simulink model "SiMoDronesBebopRos_student"  (R2021a)
settings: Solver=FixedStepAuto  StartTime=0  StopTime=35  FixedStep=0.005  MaxStep=1e-3  MinStep=5e-5  RelTol=1e-5  AbsTol=1e-5
StopFcn:
  | %data_bebop;
  | save_and_plot_data
values from neighbouring files (symbols this model uses):
  aero =     [test1_p1.mat]    (also in test2_P2.mat; test3_pd.mat; test4_lat.mat; xtest4_lat.mat)
  controlGains =     [test1_p1.mat]    (also in test2_P2.mat; test3_pd.mat; test4_lat.mat; xtest4_lat.mat)
  drone =     [test1_p1.mat]    (also in test2_P2.mat; test3_pd.mat; test4_lat.mat; xtest4_lat.mat)
  init_state =     [test1_p1.mat]    (also in test2_P2.mat; test3_pd.mat; test4_lat.mat; xtest4_lat.mat)
  K = place(A,B,P0)    [Control.m]    (also in test1_p1.mat = [0.637104994903 0.356778797146]; test2_P2.mat = [0.637104994903 0.356778797146]; test3_pd.mat = [0.637104994903 0.356778797146]; test4_lat.mat = [0.637104994903 0.356778797146])
  Kd = 3.806    [Control.m]    (also in test1_p1.mat = 5.726; test2_P2.mat = 5.726; test3_pd.mat = 5.726; test4_lat.mat = 5.726)
  Kdd = 2*sg*om*tau-1    (= 0.98)    [Control.m]    (also in test1_p1.mat = 1.509; test2_P2.mat = 1.509; test3_pd.mat; test4_lat.mat = 1.509)
  Ki = 37.39    [Control.m]    (also in test1_p1.mat = 83.71; test2_P2.mat = 83.71; test3_pd.mat = 83.71; test4_lat.mat = 83.71)
  Kp = 25.23    [Control.m]    (also in test1_p1.mat = 43.79; test2_P2.mat = 43.79; test3_pd.mat = 43.79; test4_lat.mat = 43.79)
  Kp1 = 4    [Control.m]    (also in test1_p1.mat; test2_P2.mat; test3_pd.mat; test4_lat.mat)
  Kp2 = 5.2071    [Control.m]    (also in test1_p1.mat; test2_P2.mat; test3_pd.mat; test4_lat.mat)
  Kpd = tau*om^2    (= 6.0612244898)    [Control.m]    (also in test1_p1.mat = 12.82; test2_P2.mat = 12.82; test3_pd.mat; test4_lat.mat = 12.82)
  measure =     [test1_p1.mat]    (also in test2_P2.mat; test3_pd.mat; test4_lat.mat; xtest4_lat.mat)
  motor =     [test1_p1.mat]    (also in test2_P2.mat; test3_pd.mat; test4_lat.mat; xtest4_lat.mat)
  N = K1    [Control.m]    (also in test1_p1.mat = 0.637104994903; test2_P2.mat = 0.637104994903; test3_pd.mat = 0.637104994903; test4_lat.mat = 0.637104994903)
  tau = 0.33    [Control.m]    (also in test1_p1.mat; test2_P2.mat; test3_pd.mat; test4_lat.mat)
  Te = Ts_optitrack    (= 0.02)    [Startup_bebop_ros.m]    (also in test1_p1.mat; test2_P2.mat; test3_pd.mat; test4_lat.mat)
  Te_topics_empty = 0.1    [Startup_bebop_ros.m]    (also in test1_p1.mat; test2_P2.mat; test3_pd.mat; test4_lat.mat)
  Ts_bebop = 5e-3    (= 0.005)    [Startup_bebop_ros.m]    (also in test1_p1.mat; test2_P2.mat; test3_pd.mat; test4_lat.mat)
  Ts_bebop_feedback = 2e-1    (= 0.2)    [Startup_bebop_ros.m]    (also in test1_p1.mat; test2_P2.mat; test3_pd.mat; test4_lat.mat)
  Ts_optitrack = 2e-2    (= 0.02)    [Startup_bebop_ros.m]    (also in test1_p1.mat; test2_P2.mat; test3_pd.mat; test4_lat.mat)
undefined symbols (not defined in the file or in its folder): Angular, DiscIntNeverNeededParam, gcbh, Linear, sigbuilder_block, sldros_modeswitch
libraries: robotlib x15, simulink x9, pid_lib x8, vrlib x5, lib_isae_drones x4, aerolibanimutils x2, sharedtransform x2, aerolibobsolete x1, drones x1
(part 1 of 3)
Description:
  | SiMoDronesBE is an simulation environnement for ISAE drones dedicaded at the parrot + px4 bord drone.
settings Model: xpc_rtwmakecfg_data=_xpcnblib__xpcetherlib__xpcether8255xlib__xpcetherGbElib__xpciplib_  ExtModeTrigDuration=300000  Creator=Francois Defay  LastModifiedBy=ak.sharma
settings Model: ModifiedHistory=|
  | - Modification of measurement block and visualisation
  | - Some limitations of PWM have been added on the motor
settings SolverCC: AutoScaleAbsTol=off  ZeroCrossAlgorithm=Adaptive  AlgebraicLoopSolver=TrustRegion  AutoInsertRateTranBlk=on  InsertRTBMode=Always
settings DataIOCC: SaveFormat=StructureWithTime  SaveOutput=off  DSMLogging=off  SaveTime=off  ReturnWorkspaceOutputs=off
settings OptimizationCC: BlockReduction=off  BufferReuse=off  ExpressionDepthLimit=2147483647  LifeSpan=inf
settings DebuggingCC: AlgebraicLoopMsg=none  UnderspecifiedInitializationDetection=Classic  MergeDetectMultiDrivingBlocksExec=none  IgnoredZcDiagnostic=none  MultiTaskDSMMsg=warning  UnconnectedInputMsg=none  UnconnectedOutputMsg=none  UnconnectedLineMsg=none  AllowSymbolicDim=off  StateNameClashWarn=warning  SFUnexpectedBacktrackingDiag=warning  SFNoUnconditionalDefaultTransitionDiag=warning  SFExecutionAtInitializationDiag=none  SFMachineParentedDataDiag=warning  ArithmeticOperatorsInVariantConditions=warning
settings HardwareCC: TargetBitPerLong=64  TargetBitPerPointer=64  TargetIntDivRoundTo=Zero  TargetEndianess=LittleEndian  TargetWordSize=64  TargetHWDeviceType=Intel->x86-64
settings ModelReferenceCC: PropagateSignalLabelsOutOfModel=off
settings SFSimCC: SimUseLocalCustomCode=off  CustomCodeUndefinedFunction=UseInterfaceOnly
settings RTWCC: Description=Simulink Desktop Real-Time  SystemTargetFile=sldrt.tlc  TemplateMakefile=sldrt.tmf  RTWUseLocalCustomCode=off  RTWCompilerOptimization=on
settings CodeAppCC: MaxIdLength=95  StateflowObjectComments=on
settings SimulinkDesktopRealTimeCC: TargetPreCompLibLocation=C:\Program Files\MATLAB\R2021a\toolbox\sldrt\lib\win64  TargetLangStandard=C89/C90 (ANSI)  SupportVariableSizeSignals=off
settings ConfigComp: CovMetricSettings=dw  CovSaveCumulativeToWorkspaceVar=on  CovSaveSingleToWorkspaceVar=on  CovExternalEMLEnable=off
settings SimscapeCC: SimscapeNormalizeSystem=off
settings ConfigurationSet: Description=SimMechanics 2G
settings ExplorerConfigSet: SimMechanicsOpenEditorOnUpdate=off

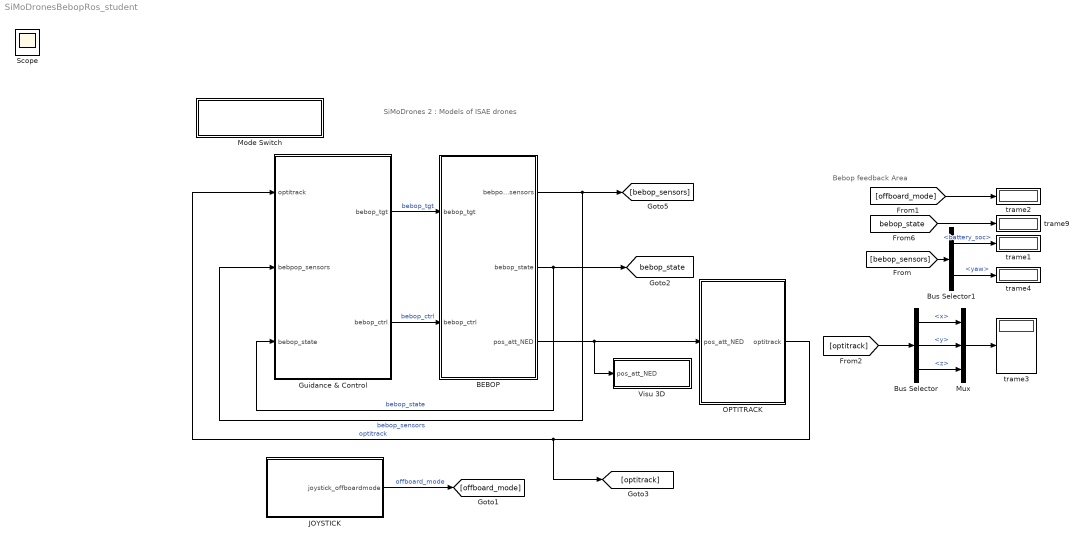
== system SiMoDronesBebopRos_student ==
  note: SiMoDrones 2 : Models of ISAE drones
  note: Bebop feedback Area
   trame{1..4,9} (5 alike) : Display
  BEBOP : Subsystem
  Bus Selector : BusSelector  OutputSignals=x,y,z
  Bus Selector1 : BusSelector  OutputSignals=battery_soc,yaw
  "Guidance & Control " : Subsystem
  JOYSTICK : Subsystem  Variant=on
  Mode Switch : Subsystem  LoadFcn=sldros_modeswitch(gcbh, false)  mask(Mode Switch){}
      settings: OpenFcn=sldros_modeswitch(gcbh, true)
      mask Display: text(0.5,0.8,'Simulation Mode', 'horizontalAlignment','center');text(0.5,0.5,'_{_{Switch To\newline Experiment Mode}}', 'horizontalAlignment','center','texmode','on');
  Mux : Mux  Inputs=3
  OPTITRACK : Subsystem  Variant=on
  Visu 3D : Subsystem  Variant=on
  Scope : Scope
  tag scope: bebop_state=global
  wires:
  Mux/1 -> " trame3"/1
  [bebop_state] -> " trame9"/1
  [offboard_mode] -> " trame2"/1
  OPTITRACK/1(optitrack) -> "Guidance & Control "/1(optitrack), [optitrack]  "optitrack"
  [optitrack] -> Bus Selector/1
  Bus Selector/1 -> Mux/1  "<x>"
  Bus Selector/2 -> Mux/2  "<y>"
  Bus Selector/3 -> Mux/3  "<z>"
  [bebop_sensors] -> Bus Selector1/1
  Bus Selector1/1 -> " trame1"/1  "<battery_soc>"
  Bus Selector1/2 -> " trame4"/1  "<yaw>"
  JOYSTICK/1(joystick_offboardmode) -> [offboard_mode]  "offboard_mode"
  BEBOP/2(bebop_state) -> [bebop_state], "Guidance & Control "/3(bebop_state)  "bebop_state"
  "Guidance & Control "/1(bebop_tgt) -> BEBOP/1(bebop_tgt)  "bebop_tgt"
  "Guidance & Control "/2(bebop_ctrl) -> BEBOP/2(bebop_ctrl)  "bebop_ctrl"
  BEBOP/1("bebpop_sensors ") -> [bebop_sensors], "Guidance & Control "/2("bebpop_sensors ")  "bebop_sensors"
  BEBOP/3(pos_att_NED) -> Visu 3D/1(pos_att_NED), OPTITRACK/1(pos_att_NED)

== system SiMoDronesBebopRos_student/BEBOP ==
  bebop_tgt : Inport
  bebop_ctrl : Inport  Port=2
  Bebop Control : Subsystem  Variant=on
  "Measurement block " : Subsystem  Variant=on
  Model : Subsystem  Variant=on
  "bebpop_sensors " : Outport  VectorParamsAs1DForOutWhenUnconnected=off
  bebop_state : Outport  Port=2  VectorParamsAs1DForOutWhenUnconnected=off
  pos_att_NED : Outport  Port=3  VectorParamsAs1DForOutWhenUnconnected=off
  wires:
  Bebop Control/1(pwm_tgt) -> Model/1(pwm_tgt)
  Model/1(pos_att_NED) -> pos_att_NED/1, "Measurement block "/1(pos_att_NED)
  Model/2(batt_info) -> "Measurement block "/2(batt_info)
  "Measurement block "/1(bebop_sensors) -> "bebpop_sensors "/1
  bebop_ctrl/1 -> Bebop Control/2(bebop_ctrl)
  bebop_tgt/1 -> Bebop Control/1(bebop_tgt)
  Bebop Control/2(bebop_state) -> bebop_state/1

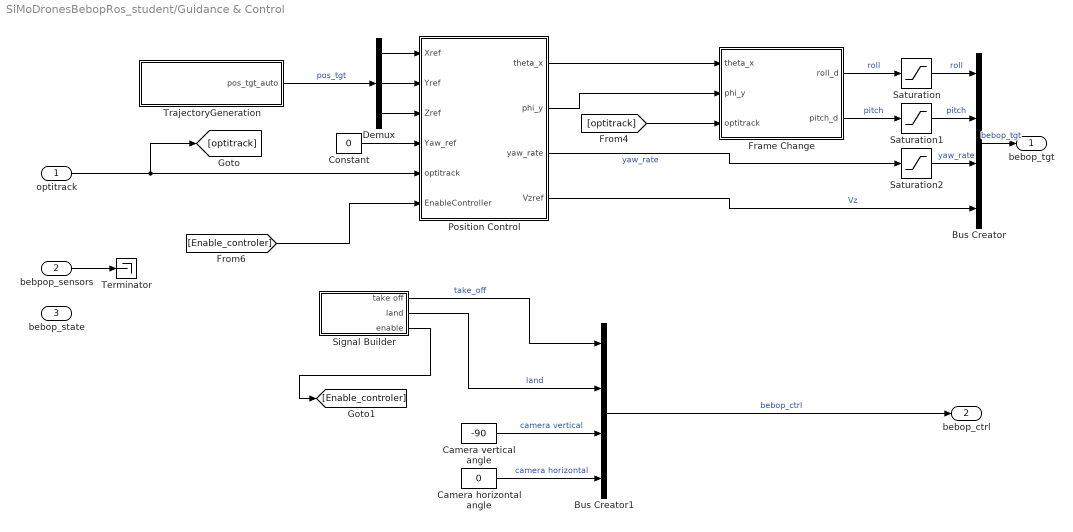
== system SiMoDronesBebopRos_student/Guidance & Control  ==
  optitrack : Inport
  "bebpop_sensors " : Inport  Port=2
  bebop_state : Inport  Port=3
  Bus Creator : BusCreator  Inputs=4  OutDataTypeStr=Bus: BUS_bebop_tgt
  Bus Creator1 : BusCreator  Inputs=4  OutDataTypeStr=Bus: BUS_bebop_ctrl
      settings: InheritFromInputs=off
  Camera horizontal angle : Constant  Value=0  SampleTime=0.02
  Camera vertical angle : Constant  Value=-90  SampleTime=0.02
  Constant : Constant  Value=0  SampleTime=0.02
  Demux : Demux  Outputs=3
  Frame Change : Subsystem
  Position Control : Subsystem
  Saturation : Saturate  UpperLimit=controlGains.pitch.anglemax  LowerLimit=-controlGains.pitch.anglemax
  Saturation1 : Saturate  UpperLimit=controlGains.roll.anglemax  LowerLimit=-controlGains.roll.anglemax
  Saturation2 : Saturate  UpperLimit=controlGains.psi.ratemax  LowerLimit=-controlGains.psi.ratemax
  Signal Builder : Subsystem  Tag=STV Subsys  LoadFcn=sigbuilder_block('load');  StartFcn=sigbuilder_block('start');  StopFcn=sigbuilder_block('stop');  ClipboardFcn=sigbuilder_block('clipboard');  mask(Sigbuilder block){tuvar=[0:10]}
      mask help: Simulink:masks:SigbuilderBlock_MD
      mask init:
      | if ~strcmp(get_param(bdroot(gcbh),'SimulationStatus'),'stopped') tuvar = sigbuilder_block('maskInit'); end
      settings: CopyFcn=sigbuilder_block('copy');  DeleteFcn=sigbuilder_block('delete');  ModelCloseFcn=sigbuilder_block('modelClose');  PreSaveFcn=sigbuilder_block('preSave');  PauseFcn=sigbuilder_block('pause');  ContinueFcn=sigbuilder_block('continue');  NameChangeFcn=sigbuilder_block('namechange');  OpenFcn=sigbuilder_block('open',[651 216 550.5 399.75 ]);  CloseFcn=sigbuilder_block('close');
      mask Display: plot(0, 0, 100, 100,[2, 2, 32, 32, 2], [68, 8, 8, 68, 68],[32, 2], [38, 38], [32, 19, 2],[53, 60, 44], [32, 17, 17, 2],[16, 16, 31, 31]);txt = getActiveGroup(gcbh);text(2, 100, txt,'verticalAlignment', 'top');
  Terminator : Terminator
  TrajectoryGeneration : Subsystem
  bebop_tgt : Outport  VectorParamsAs1DForOutWhenUnconnected=off
  bebop_ctrl : Outport  Port=2  VectorParamsAs1DForOutWhenUnconnected=off
  wires:
  Position Control/1(theta_x) -> Frame Change/1(theta_x)
  Position Control/2(phi_y) -> Frame Change/2(phi_y)
  Demux/1 -> Position Control/1(Xref)
  Demux/2 -> Position Control/2(Yref)
  Constant/1 -> Position Control/4(Yaw_ref)
  Demux/3 -> Position Control/3(Zref)
  [optitrack] -> Frame Change/3(optitrack)
  "bebpop_sensors "/1 -> Terminator/1
  Bus Creator/1 -> bebop_tgt/1  "bebop_tgt"
  Position Control/4(Vzref) -> Bus Creator/4  "Vz"
  Frame Change/1(roll_d) -> Saturation/1  "roll"
  Position Control/3(yaw_rate) -> Saturation2/1  "yaw_rate"
  Frame Change/2(pitch_d) -> Saturation1/1  "pitch"
  Camera vertical angle/1 -> Bus Creator1/3  "camera vertical"
  Camera horizontal angle/1 -> Bus Creator1/4  "camera horizontal"
  Bus Creator1/1 -> bebop_ctrl/1  "bebop_ctrl"
  TrajectoryGeneration/1(pos_tgt_auto) -> Demux/1  "pos_tgt"
  optitrack/1 -> Position Control/5(optitrack), [optitrack]
  Saturation/1 -> Bus Creator/1  "roll"
  Saturation1/1 -> Bus Creator/2  "pitch"
  Saturation2/1 -> Bus Creator/3  "yaw_rate"
  [Enable_controler] -> Position Control/6(EnableController)
  Signal Builder/3(enable) -> [Enable_controler]
  Signal Builder/2(land) -> Bus Creator1/2  "land"
  Signal Builder/1(take off) -> Bus Creator1/1  "take_off"

== system SiMoDronesBebopRos_student/JOYSTICK ==
  "Measure " : Subsystem  VariantControl=SIMULATION_MODE
  ROS link + Measure : Subsystem  VariantControl=EXPERIMENT_MODE
  joystick_offboardmode : Outport  VectorParamsAs1DForOutWhenUnconnected=off

== system SiMoDronesBebopRos_student/Mode Switch ==
  mode : Constant  Value=0

== system SiMoDronesBebopRos_student/OPTITRACK ==
  pos_att_NED : Inport
  "Measure " : Subsystem  VariantControl=SIMULATION_MODE
  ROS link + Measure : Subsystem  VariantControl=EXPERIMENT_MODE
  optitrack : Outport  VectorParamsAs1DForOutWhenUnconnected=off

== system SiMoDronesBebopRos_student/Visu 3D ==
  pos_att_NED : Inport
  3D disabled : Subsystem  VariantControl=EXPERIMENT_MODE
  Simulink 3D : Subsystem  VariantControl=SIMULATION_MODE

== system SiMoDronesBebopRos_student/BEBOP/Bebop Control ==
  bebop_tgt : Inport
  bebop_ctrl : Inport  Port=2
  Inner Loop (Parrot) : Subsystem  VariantControl=SIMULATION_MODE
  Udp send : Subsystem  VariantControl=EXPERIMENT_MODE
  pwm_tgt : Outport  VectorParamsAs1DForOutWhenUnconnected=off
  bebop_state : Outport  Port=2  VectorParamsAs1DForOutWhenUnconnected=off

== system SiMoDronesBebopRos_student/BEBOP/Measurement block  ==
  pos_att_NED : Inport  OutDataTypeStr=Bus: BUS_bebop_pos_att
  batt_info : Inport  Port=2
  "Measure " : Subsystem  VariantControl=SIMULATION_MODE
  ROS link + Measure : Subsystem  VariantControl=EXPERIMENT_MODE
  bebop_sensors : Outport  OutDataTypeStr=Bus: BUS_bebop_sensors  VectorParamsAs1DForOutWhenUnconnected=off

== system SiMoDronesBebopRos_student/BEBOP/Model ==
  pwm_tgt : Inport
  Model : Subsystem  VariantControl=SIMULATION_MODE
  Model disabled : Subsystem  VariantControl=EXPERIMENT_MODE
  pos_att_NED : Outport  OutDataTypeStr=Bus: BUS_bebop_pos_att  VectorParamsAs1DForOutWhenUnconnected=off
  batt_info : Outport  Port=2  VectorParamsAs1DForOutWhenUnconnected=off

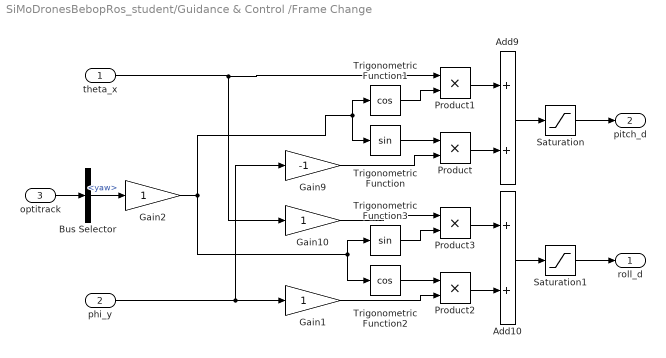
== system SiMoDronesBebopRos_student/Guidance & Control /Frame Change ==
  theta_x : Inport
  phi_y : Inport  Port=2
  optitrack : Inport  Port=3
  Add10 : Sum
  Add9 : Sum
  Bus Selector : BusSelector  OutputSignals=yaw
  Gain1 : Gain
  Gain10 : Gain
  Gain2 : Gain
  Gain9 : Gain  Gain=-1
  Product{,1..3} (4 alike) : Product
  Saturation : Saturate  UpperLimit=0.3  LowerLimit=-0.3
  Saturation1 : Saturate  UpperLimit=0.3  LowerLimit=-0.3
  Trigonometric Function : Trigonometry
  Trigonometric Function1 : Trigonometry  Operator=cos
  Trigonometric Function2 : Trigonometry  Operator=cos
  Trigonometric Function3 : Trigonometry
  roll_d : Outport  VectorParamsAs1DForOutWhenUnconnected=off
  pitch_d : Outport  Port=2  VectorParamsAs1DForOutWhenUnconnected=off
  wires:
  Gain2/1 -> Trigonometric Function/1, Trigonometric Function1/1, Trigonometric Function2/1, Trigonometric Function3/1
  theta_x/1 -> Product1/1, Gain10/1
  Saturation/1 -> pitch_d/1
  phi_y/1 -> Gain9/1, Gain1/1
  Saturation1/1 -> roll_d/1
  Add9/1 -> Saturation/1
  Product/1 -> Add9/2
  Product1/1 -> Add9/1
  Trigonometric Function/1 -> Product/1
  Trigonometric Function1/1 -> Product1/2
  Add10/1 -> Saturation1/1
  Product2/1 -> Add10/2
  Product3/1 -> Add10/1
  Trigonometric Function2/1 -> Product2/1
  Trigonometric Function3/1 -> Product3/2
  Gain9/1 -> Product/2
  Gain10/1 -> Product3/1
  optitrack/1 -> Bus Selector/1
  Bus Selector/1 -> Gain2/1  "<yaw>"
  Gain1/1 -> Product2/2

== system SiMoDronesBebopRos_student/Guidance & Control /Position Control ==
  Xref : Inport
  Yref : Inport  Port=2
  Zref : Inport  Port=3
  Yaw_ref : Inport  Port=4
  optitrack : Inport  Port=5
  EnableController : Inport  Port=6
  Bus Selector1 : BusSelector  OutputSignals=x,Vx,y,Vy,z,yaw,Vz
  "Control x " : Subsystem
  Control y : Subsystem
  Control yaw : Subsystem
  Control z : Subsystem
  theta_x : Outport  VectorParamsAs1DForOutWhenUnconnected=off
  phi_y : Outport  Port=2  VectorParamsAs1DForOutWhenUnconnected=off
  yaw_rate : Outport  Port=3  VectorParamsAs1DForOutWhenUnconnected=off
  Vzref : Outport  Port=4  VectorParamsAs1DForOutWhenUnconnected=off
  wires:
  "Control x "/1(theta_x) -> theta_x/1  "theta_x"
  Bus Selector1/1 -> "Control x "/2(X)  "<x>"
  Control y/1(phi_y) -> phi_y/1  "phi_y"
  Control z/1(VZref) -> Vzref/1  "Vz"
  Bus Selector1/2 -> "Control x "/3("VX ")  "<Vx>"
  Xref/1 -> "Control x "/1(Xref)
  optitrack/1 -> Bus Selector1/1
  Bus Selector1/5 -> Control z/3(Z)  "<z>"
  Control yaw/1(yaw_rate) -> yaw_rate/1
  Bus Selector1/3 -> Control y/2(Y)  "<y>"
  Bus Selector1/4 -> Control y/3("VY ")  "<Vy>"
  Yaw_ref/1 -> Control yaw/1(yaw_ref)
  Bus Selector1/6 -> Control yaw/2(yaw)  "<yaw>"
  Yref/1 -> Control y/1(Yref)
  Zref/1 -> Control z/1(Zref)
  EnableController/1 -> "Control x "/Enable, Control y/Enable, Control yaw/Enable, Control z/Enable
  Bus Selector1/7 -> Control z/2(Vz)  "<Vz>"

== system SiMoDronesBebopRos_student/Guidance & Control /Signal Builder ==
  Demux : Demux  Tag=STV Demux  Outputs=3
      settings: DisplayOption=none
  FromWs : FromWorkspace  Tag=STV FromWs  VariableName=tuvar  SampleTime=0.02
      SigBuilderData=|
      | common.afterFinalStr = 'Extrapolate'
      | common.sampleTime = '0.02'
      | dataSet.timeRange = [0 35]
      | dataSet.name = 'Group 1'
      | sbobj.Groups.Name = 'Group 1'
      | sbobj.Groups.Signals(1).Name = 'take off'
      | sbobj.Groups.Signals(1).XData = [0 0.8 0.8 8 8 35]
      | sbobj.Groups.Signals(1).YData = [0 0 1 1 0 0]
      | sbobj.Groups.Signals(2).Name = 'land'
      | sbobj.Groups.Signals(2).XData = [0 30 30 35]
      | sbobj.Groups.Signals(2).YData = [0 0 1 1]
      | sbobj.Groups.Signals(3).Name = 'enable'
      | sbobj.Groups.Signals(3).XData = [0 8 8 30 30 35]
      | sbobj.Groups.Signals(3).YData = [0 0 1 1 0 0]
      | sbobj.Groups.TimeRange = [0 35]
  take off : Outport  Tag=STV Outport
  land : Outport  Tag=STV Outport  Port=2
  enable : Outport  Tag=STV Outport  Port=3
  wires:
  Demux/1 -> take off/1
  FromWs/1 -> Demux/1
  Demux/2 -> land/1
  Demux/3 -> enable/1

== system SiMoDronesBebopRos_student/Guidance & Control /TrajectoryGeneration ==
  Mux : Mux  Inputs=3
  Step : Step  Time=15  Before=-1.5  After=-2  SampleTime=0.02
  Step1 : Step  Time=15  After=-0.2  SampleTime=0.02
  Step2 : Step  Time=10  After=-0.2  SampleTime=0.02
  Step3 : Step  Time=25  After=0.2  SampleTime=0.02
  Step4 : Step  Time=20  After=0.2  SampleTime=0.02
  Sum1 : Sum  Inputs=|++
  Sum2 : Sum  Inputs=|++
  pos_tgt_auto : Outport  VectorParamsAs1DForOutWhenUnconnected=off
  wires:
  Mux/1 -> pos_tgt_auto/1
  Step2/1 -> Sum1/1  "xref"
  Step4/1 -> Sum1/2  "xref"
  Sum1/1 -> Mux/1
  Sum2/1 -> Mux/2
  Step/1 -> Mux/3  "zref"
  Step3/1 -> Sum2/2  "yref"
  Step1/1 -> Sum2/1  "yref"

== system SiMoDronesBebopRos_student/JOYSTICK/Measure  ==
  Constant : Constant  SampleTime=Te
  joystick_offboardmode : Outport  VectorParamsAs1DForOutWhenUnconnected=off
  wires:
  Constant/1 -> joystick_offboardmode/1

== system SiMoDronesBebopRos_student/JOYSTICK/ROS link + Measure ==
  UDP link : Subsystem
  joystick_offboardmode : Outport  VectorParamsAs1DForOutWhenUnconnected=off
  wires:
  UDP link/1(joystick_offboardmode) -> joystick_offboardmode/1

== system SiMoDronesBebopRos_student/OPTITRACK/Measure  ==
  pos_att_NED : Inport
  optitrack_ : Subsystem
  optitrack : Outport  OutDataTypeStr=Bus: BUS_optitrack  VectorParamsAs1DForOutWhenUnconnected=off
  wires:
  optitrack_/1(optitrack_) -> optitrack/1
  pos_att_NED/1 -> optitrack_/1(pos_att_NED)

== system SiMoDronesBebopRos_student/OPTITRACK/ROS link + Measure ==
  UDP link : Subsystem
  optitrack : Outport  OutDataTypeStr=Bus: BUS_optitrack  VectorParamsAs1DForOutWhenUnconnected=off
  wires:
  UDP link/1(optitrack) -> optitrack/1

== system SiMoDronesBebopRos_student/Visu 3D/3D disabled ==

== system SiMoDronesBebopRos_student/Visu 3D/Simulink 3D ==
  pos_att_NED : Inport
  Coordinate Transformations : Subsystem
  Simulation Pace : aerolibanimutils/Simulation Pace  SimulationPace=10  SleepMode=MATLAB Thread  OutputPaceError=off  SampleTime=Te
      settings: AttributesFormatString=%<SimulationPace> sec/sec
  VR Sink : vrlib/VR Sink  InstantiateOnLoad=on  SampleTime=0.1  ViewEnable=on  RemoteChange=off  RemoteView=off  FieldsWritten=Camera_Follow.rotation.4.1.1.double#Camera_Follow.translation.3.1.1.double#Copter.rotation.4.1.1.double#Copter.translation.3.1.1.double  WorldFileName=Visu/ArduCopter.wrl  WorldDescription=VR Arducopter  AutoView=off  VideoDimensions=[]  AllowVariableSize=off
  wires:
  Coordinate Transformations/4(position) -> VR Sink/4
  Coordinate Transformations/3(orientation) -> VR Sink/3
  Coordinate Transformations/2(CameraFollowTranslation) -> VR Sink/2
  Coordinate Transformations/1(CameraFollowRotation) -> VR Sink/1
  pos_att_NED/1 -> Coordinate Transformations/1(pos_att_NED)

== system SiMoDronesBebopRos_student/BEBOP/Bebop Control/Inner Loop (Parrot) ==
  bebop_tgt : Inport  OutDataTypeStr=Bus: BUS_bebop_tgt
  bebop_ctrl : Inport  Port=2
  Bebop onboard control : Subsystem  VariantControl=SIMULATION_SIMULINK  mask(PX4 attitude controller){thetaKP=controlGains.pitch.thetaKP, thetaKI=controlGains.pitch.thetaKI, thetaKD=controlGains.pitch.thetaKD, thetaKDD=controlGains.pitch.thetaKDD, pitchmax=controlGains.pitch.anglemax, phiKP=controlGains.roll.phiKP, phiKI=controlGains.roll.phiKI, phiKD=controlGains.roll.phiKD, phiKDD=controlGains.roll.phiKDD, phimax=controlGains.roll.anglemax, altiKP=controlGains.altitude.KP, altiKI=controlGains.altitude.KI, altiKD=controlGains.altitude.KD, altiVzmax=controlGains.altitude.VZmax}
      mask prompts: thetaKP "Proportional gain"; thetaKI "Integral gain"; thetaKD "Derivative gain"; thetaKDD "Feed forward gain"; pitchmax "Max angle (rad)"; phiKP "Proportional gain"; phiKI "Integral gain"; phiKD "Derivative gain"; phiKDD "Feed forward gain"; phimax "Max angle (rad)"; altiKP "Proportional gain"; altiKI "Integral gain"; altiKD "Derivative gain"; altiVzmax "Max Vertical speed(rad)"
      mask DialogControl Container4 Prompt: Pitch control
      mask DialogControl Container5 Prompt: Roll control
      mask DialogControl Container6 Prompt: Vertical control
  Mixer_Quad_X : Subsystem  mask(Mixer Quad X){}
      mask help:
      | Mixer used by a PX4 configured with a Quad X airframe.
      |
      | It takes in the the actuators target (normalized roll, pitch, yaw [-1..1], thrust [0..1]) and mixes them with the Quad X mixer matrix into 4 motors PWM ([0..1]).
      mask DialogControl Container2 Prompt: Parameters
  pwm_tgt : Outport  VectorParamsAs1DForOutWhenUnconnected=off
  bebop_state : Outport  Port=2  VectorParamsAs1DForOutWhenUnconnected=off
  wires:
  [bebop_sensors_local] -> Bebop onboard control/3(bebop_sensors)
  Bebop onboard control/1(actuator_target) -> Mixer_Quad_X/1(actuators_tgt)
  Mixer_Quad_X/1(pwm_out) -> pwm_tgt/1
  bebop_tgt/1 -> Bebop onboard control/1(bebop_tgt)
  bebop_ctrl/1 -> Bebop onboard control/2(bebop_ctrl)
  Bebop onboard control/2(bebop_state) -> bebop_state/1

== system SiMoDronesBebopRos_student/BEBOP/Bebop Control/Udp send ==
  bebop_tgt : Inport
  bebop_ctrl : Inport  Port=2
  Bus Selector : BusSelector  OutputSignals=camera_vertical,camera_horizontal,takeoff,land
  Bus Selector3 : BusSelector  OutputSignals=pitch,roll,yaw_rate,Vz
  Bus Selector5 : BusSelector  OutputSignals=Data
  NED attitude to ENU linear : Subsystem
  Simulation Pace : aerolibanimutils/Simulation Pace  SimulationPace=1  SleepMode=MATLAB Thread  OutputPaceError=off  SampleTime=Te
      settings: AttributesFormatString=%<SimulationPace> sec/sec
  Subscribe5 : robotlib/Subscribe  topicSource=Select from ROS network  topic=/bebop/state  messageType=std_msgs/Float64  SampleTime=Ts_bebop_feedback  legacyBusStruct=off  messageQueueLength=1
      link override SourceBlock: ROSTopic=/bebop/state  ROSMessageType=std_msgs/Float64  SLBusName=SL_Bus_SiMoDronesBebopRos_student_std_msgs_Float64  ModelName=SiMoDronesBebopRos_student  BlockId=Sub_SiMoDronesBebopRos_student_14953
  Topics : Subsystem
  bebop_state : Outport  VectorParamsAs1DForOutWhenUnconnected=off
  wires:
  bebop_tgt/1 -> Bus Selector3/1
  [Vz_tgt] -> NED attitude to ENU linear/3(<vz>)
  Bus Selector3/3 -> NED attitude to ENU linear/4(<body_yaw_rate>)  "<yaw_rate>"
  Bus Selector3/2 -> NED attitude to ENU linear/2(<roll>)  "<roll>"
  Bus Selector3/1 -> NED attitude to ENU linear/1(<pitch>)  "<pitch>"
  NED attitude to ENU linear/1(Out1) -> Topics/1(linear.X)
  NED attitude to ENU linear/2(Out2) -> Topics/2(Linera.Y)
  NED attitude to ENU linear/3(Out3) -> Topics/3(linera.Z)
  NED attitude to ENU linear/4(Out4) -> Topics/4(Angular.Z)
  Bus Selector/1 -> Topics/5(Camera.vertical angle)  "<camera_vertical>"
  Bus Selector/3 -> Topics/7(Order.takeOff)  "<takeoff>"
  Bus Selector/4 -> Topics/8(Order.Land)  "<land>"
  bebop_ctrl/1 -> Bus Selector/1
  Bus Selector/2 -> Topics/6(Camera.horizontal angle)  "<camera_horizontal>"
  Bus Selector3/4 -> [Vz_tgt]  "<Vz>"
  Subscribe5/2 -> Bus Selector5/1
  Bus Selector5/1 -> bebop_state/1  "<Data>"

== system SiMoDronesBebopRos_student/BEBOP/Measurement block /Measure  ==
  pos_att_NED : Inport  OutDataTypeStr=Bus: BUS_bebop_pos_att
  batt_info : Inport  Port=2
  bebop : Subsystem
  bebop_sensors : Outport  OutDataTypeStr=Bus: BUS_bebop_sensors  VectorParamsAs1DForOutWhenUnconnected=off
  wires:
  bebop/1(bebop_sensors) -> bebop_sensors/1
  pos_att_NED/1 -> bebop/1(pos_att_NED)  "pos_att_NED"
  batt_info/1 -> bebop/2(batt)

== system SiMoDronesBebopRos_student/BEBOP/Measurement block /ROS link + Measure ==
  UDP link : Subsystem
  bebop_sensors : Outport  OutDataTypeStr=Bus: BUS_bebop_sensors  VectorParamsAs1DForOutWhenUnconnected=off
  wires:
  UDP link/1(bebop_sensors) -> bebop_sensors/1

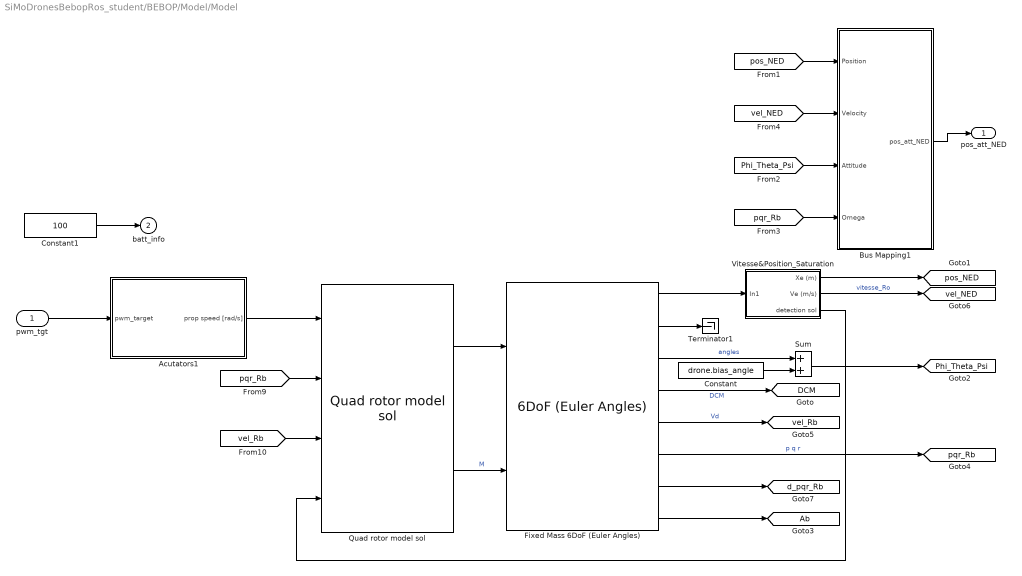
== system SiMoDronesBebopRos_student/BEBOP/Model/Model ==
  pwm_tgt : Inport
  Acutators1 : Subsystem
  Bus Mapping1 : Subsystem
  Constant : Constant  Value=drone.bias_angle
  Constant1 : Constant  Value=100  SampleTime=0
  Fixed Mass 6DoF (Euler Angles) : aerolibobsolete/6DoF (Euler Angles)  units=Metric (MKS)  mtype=Fixed  rep=Euler Angles  xme_0=init_state.Pterre0  Vm_0=init_state.Vuvw0  eul_0=init_state.Angles0  pm_0=init_state.pqr0  mass_0=drone.mtot  mass_e=0  mass_f=0  inertia=drone.Itot  inertia_e=eye(3)  inertia_f=eye(3)  k_quat=1.0
      settings: SourceProductBaseCode=AE
  Quad rotor model sol : drones/Quad rotor model sol  Pw=motor.Pw  L=drone.lenght_arm  Mw=motor.Mw  mtot=drone.mtot  rho=aero.rho  S_drag_uvw=aero.S_trainee_uvw  C_drag=aero.C_trainee  g=aero.g  C_trainee=0  S_trainee_pqr=0
  Sum : Sum
  Terminator1 : Terminator
  Vitesse&Position_Saturation : Subsystem
  pos_att_NED : Outport  OutDataTypeStr=Bus: BUS_bebop_pos_att  VectorParamsAs1DForOutWhenUnconnected=off
  batt_info : Outport  Port=2  SampleTime=0  VectorParamsAs1DForOutWhenUnconnected=off
  tag scope: Ab=global, DCM=global, Phi_Theta_Psi=global, d_pqr_Rb=global, pos_NED=global, pqr_Rb=global, vel_NED=global, vel_Rb=global
  wires:
  Vitesse&Position_Saturation/2(Ve (m/s)) -> [vel_NED]  "vitesse_Ro"
  Fixed Mass 6DoF (Euler Angles)/8 -> [Ab]
  Fixed Mass 6DoF (Euler Angles)/5 -> [vel_Rb]  "Vd"
  Fixed Mass 6DoF (Euler Angles)/4 -> [DCM]  "DCM"
  Fixed Mass 6DoF (Euler Angles)/3 -> Sum/1  "angles"
  Fixed Mass 6DoF (Euler Angles)/1 -> Vitesse&Position_Saturation/1(In1)
  Fixed Mass 6DoF (Euler Angles)/2 -> Terminator1/1
  Fixed Mass 6DoF (Euler Angles)/6 -> [pqr_Rb]  "p q r"
  Fixed Mass 6DoF (Euler Angles)/7 -> [d_pqr_Rb]
  [pqr_Rb] -> Quad rotor model sol/2
  pwm_tgt/1 -> Acutators1/1(pwm_target)
  [pos_NED] -> Bus Mapping1/1(Position)
  [vel_NED] -> Bus Mapping1/2(Velocity)
  [pqr_Rb] -> Bus Mapping1/4(Omega)
  [Phi_Theta_Psi] -> Bus Mapping1/3(Attitude)
  Bus Mapping1/1(pos_att_NED) -> pos_att_NED/1
  Quad rotor model sol/2 -> Fixed Mass 6DoF (Euler Angles)/2  "M"
  [vel_Rb] -> Quad rotor model sol/3
  Quad rotor model sol/1 -> Fixed Mass 6DoF (Euler Angles)/1
  Sum/1 -> [Phi_Theta_Psi]
  Constant/1 -> Sum/2
  Vitesse&Position_Saturation/1(Xe (m)) -> [pos_NED]
  Vitesse&Position_Saturation/3(detection sol) -> Quad rotor model sol/4
  Acutators1/1(prop speed [rad/s]) -> Quad rotor model sol/1
  Constant1/1 -> batt_info/1

== system SiMoDronesBebopRos_student/BEBOP/Model/Model disabled ==

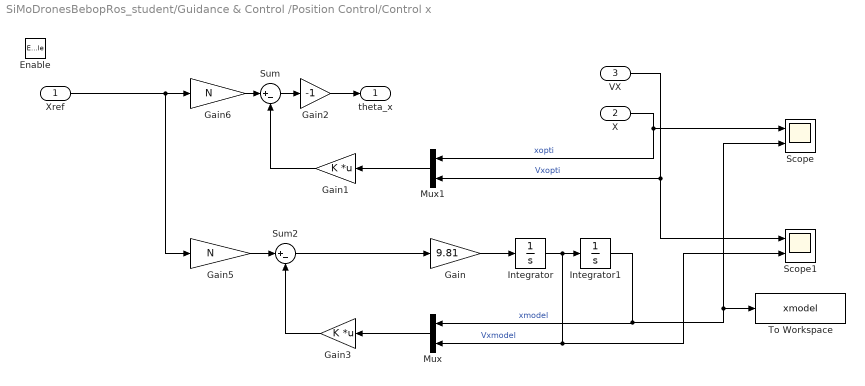
== system SiMoDronesBebopRos_student/Guidance & Control /Position Control/Control x  ==
  Xref : Inport
  X : Inport  Port=2
  "VX " : Inport  Port=3
  Enable : EnablePort
  Gain : Gain  Gain=9.81
  Gain1 : Gain  Gain=K  Multiplication=Matrix(K*u)
  Gain2 : Gain  Gain=-1
  Gain3 : Gain  Gain=K  Multiplication=Matrix(K*u)
  Gain5 : Gain  Gain=N
  Gain6 : Gain  Gain=N
  Integrator : Integrator
  Integrator1 : Integrator
  Mux : Mux  Inputs=2
  Mux1 : Mux  Inputs=2
  Scope : Scope  NumInputPorts=2
  Scope1 : Scope  NumInputPorts=2
  Sum : Sum  Inputs=|+-
  Sum2 : Sum  Inputs=|+-
  To Workspace : ToWorkspace  VariableName=xmodel  SaveFormat=Timeseries  SampleTime=-1
  theta_x : Outport  InitialOutput=0  VectorParamsAs1DForOutWhenUnconnected=off
  wires:
  X/1 -> Mux1/1, Scope/1  "xopti"
  Gain/1 -> Integrator/1
  Integrator/1 -> Scope1/2, Mux/2, Integrator1/1  "Vxmodel"
  Integrator1/1 -> To Workspace/1, Scope/2, Mux/1  "xmodel"
  Xref/1 -> Gain5/1, Gain6/1
  Gain5/1 -> Sum2/1
  Gain6/1 -> Sum/1
  Mux/1 -> Gain3/1
  Gain3/1 -> Sum2/2
  Mux1/1 -> Gain1/1
  "VX "/1 -> Mux1/2, Scope1/1  "Vxopti"
  Gain1/1 -> Sum/2
  Sum/1 -> Gain2/1
  Gain2/1 -> theta_x/1
  Sum2/1 -> Gain/1

== system SiMoDronesBebopRos_student/Guidance & Control /Position Control/Control y ==
  Yref : Inport
  Y : Inport  Port=2
  "VY " : Inport  Port=3
  Enable : EnablePort
  Gain : Gain  Gain=9.81
  Gain1 : Gain  Gain=K  Multiplication=Matrix(K*u)
  Gain2 : Gain  Gain=N
  Gain3 : Gain  Gain=K  Multiplication=Matrix(K*u)
  Gain5 : Gain  Gain=N
  Integrator : Integrator
  Integrator1 : Integrator
  Mux : Mux  Inputs=2
  Mux1 : Mux  Inputs=2
  Scope : Scope  NumInputPorts=2
  Scope1 : Scope  NumInputPorts=2
  Sum : Sum  Inputs=|+-
  Sum1 : Sum  Inputs=|+-
  To Workspace : ToWorkspace  VariableName=ymodel  SaveFormat=Timeseries  SampleTime=-1
  phi_y : Outport  InitialOutput=0  VectorParamsAs1DForOutWhenUnconnected=off
  wires:
  Yref/1 -> Gain2/1, Gain5/1
  Integrator1/1 -> To Workspace/1, Mux/1, Scope/2  "ymodel"
  Integrator/1 -> Mux/2, Scope1/2, Integrator1/1  "Vymodel"
  Gain/1 -> Integrator/1
  Y/1 -> Mux1/1, Scope/1  "yopti"
  Mux/1 -> Gain3/1
  Gain5/1 -> Sum1/1
  Gain3/1 -> Sum1/2
  Sum1/1 -> Gain/1
  Mux1/1 -> Gain1/1
  "VY "/1 -> Scope1/1, Mux1/2  "Vyopti"
  Gain1/1 -> Sum/2
  Gain2/1 -> Sum/1
  Sum/1 -> phi_y/1

== system SiMoDronesBebopRos_student/Guidance & Control /Position Control/Control yaw ==
  yaw_ref : Inport
  yaw : Inport  Port=2
  Enable : EnablePort
  Gain : Gain
  Sum : Sum  Inputs=|+-
  yaw_rate : Outport  OutputWhenDisabled=reset  InitialOutput=0  VectorParamsAs1DForOutWhenUnconnected=off
  wires:
  Sum/1 -> Gain/1
  yaw/1 -> Sum/2
  yaw_ref/1 -> Sum/1
  Gain/1 -> yaw_rate/1

== system SiMoDronesBebopRos_student/Guidance & Control /Position Control/Control z ==
  Zref : Inport
  Vz : Inport  Port=2
  Z : Inport  Port=3
  Enable : EnablePort
  Manual Switch : ManualSwitch
  Manual Switch1 : ManualSwitch
  Manual Switch2 : ManualSwitch
  P controller - 1st order system : Subsystem
  P controller - 2nd order system : Subsystem
  PD controller - 2nd order system : Subsystem
  PID controller - 2nd order system : Subsystem
  Step : Step  Commented=on  Time=15  After=-0.1  SampleTime=0.02
  VZref : Outport  OutputWhenDisabled=reset  InitialOutput=0  VectorParamsAs1DForOutWhenUnconnected=off
  wires:
  Vz/1 -> P controller - 1st order system/2(Vz), P controller - 2nd order system/2(Vz), PID controller - 2nd order system/2(Vz), PD controller - 2nd order system/2(Vz)  "Vzopti"
  Z/1 -> P controller - 1st order system/3(Z), P controller - 2nd order system/3(Z), PID controller - 2nd order system/3(Z), PD controller - 2nd order system/3(Z)  "opti"
  P controller - 1st order system/1(VZref) -> Manual Switch/1
  Manual Switch/1 -> Manual Switch1/1
  Manual Switch1/1 -> VZref/1
  Zref/1 -> PID controller - 2nd order system/1(Zref), PD controller - 2nd order system/1(Zref), P controller - 2nd order system/1(Zref), P controller - 1st order system/1(Zref)
  PD controller - 2nd order system/1(VZref) -> Manual Switch2/1
  PID controller - 2nd order system/1(VZref) -> Manual Switch2/2
  Manual Switch2/1 -> Manual Switch1/2
  P controller - 2nd order system/1(VZref) -> Manual Switch/2

== system SiMoDronesBebopRos_student/JOYSTICK/ROS link + Measure/UDP link ==
  Bus Selector7 : BusSelector  OutputSignals=Data
  MATLAB Function : MATLAB Function  TreatAsAtomicUnit=on
  Subscribe7 : robotlib/Subscribe  topicSource=Select from ROS network  topic=/mux_cmd_vel/selected  messageType=std_msgs/String  SampleTime=Te  legacyBusStruct=off  messageQueueLength=1
  joystick_offboardmode : Outport  VectorParamsAs1DForOutWhenUnconnected=off
  wires:
  Bus Selector7/1 -> MATLAB Function/1(selected_topic)  "<Data>"
  Subscribe7/2 -> Bus Selector7/1
  MATLAB Function/1(offboard) -> joystick_offboardmode/1

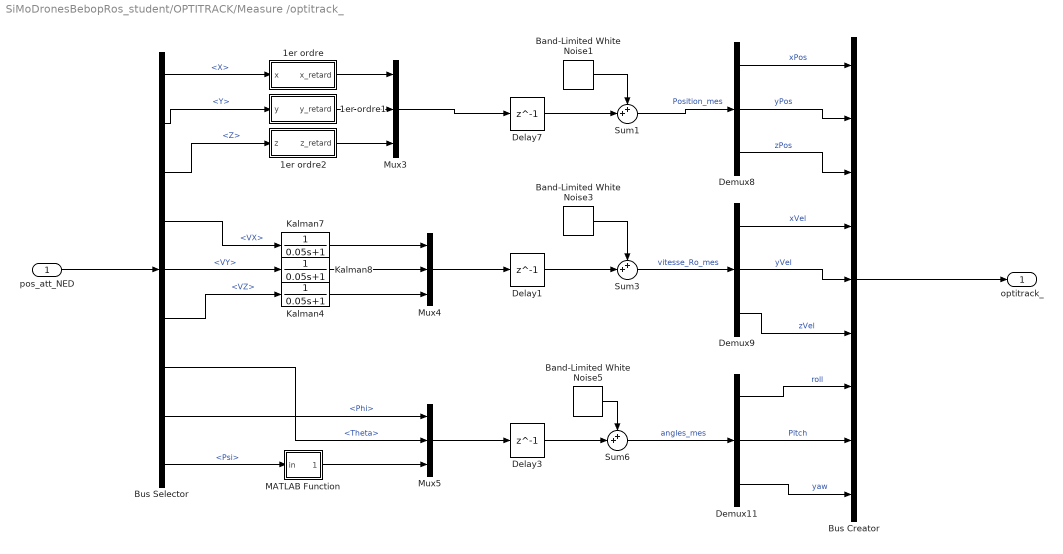
== system SiMoDronesBebopRos_student/OPTITRACK/Measure /optitrack_ ==
  pos_att_NED : Inport
  1er ordre : Subsystem  mask{tr5=0.007, K=1, init_inte=init_state.Pterre0(1)}
      mask prompts: tr5 "Tau"; K "Gain Statique"; init_inte "Initialisation 1/p"
  1er ordre1 : Subsystem  mask{tr5=0.007, K=1, init_inte=init_state.Pterre0(2)}
      mask prompts: tr5 "Tau"; K "Gain Statique"; init_inte "Initialisation 1/p"
  1er ordre2 : Subsystem  mask{tr5=0.05, K=1, init_inte=init_state.Pterre0(3)}
      mask prompts: tr5 "Tau"; K "Gain Statique"; init_inte "Initialisation 1/p"
  Band-Limited White Noise1 : simulink/Sources/Band-Limited White Noise  Cov=[measure.noise_power]  Ts=Ts_optitrack  seed=[23341]
  Band-Limited White Noise3 : simulink/Sources/Band-Limited White Noise  Cov=[measure.noise_power_vit]  Ts=Ts_optitrack  seed=[23341]
  Band-Limited White Noise5 : simulink/Sources/Band-Limited White Noise  Cov=[measure.noise_power_angles]  Ts=Ts_optitrack  seed=[23341]
  Bus Creator : BusCreator  Inputs=9  OutDataTypeStr=Bus: BUS_optitrack
      settings: InheritFromInputs=off
  Bus Selector : BusSelector  OutputSignals=X,Y,Z,VX,VY,VZ,Phi,Theta,Psi
  Delay1 : Delay  DelayLength=1  InitialCondition=init_state.Vuvw0  SampleTime=Ts_optitrack
  Delay3 : Delay  DelayLength=1  InitialCondition=init_state.Angles0  SampleTime=Ts_optitrack
  Delay7 : Delay  DelayLength=1  InitialCondition=init_state.Pterre0  SampleTime=Ts_optitrack
  Demux11 : Demux  Outputs=3
  Demux8 : Demux  Outputs=3
  Demux9 : Demux  Outputs=3
  Kalman4 : TransferFcn  Denominator=[0.05 1]
  Kalman7 : TransferFcn  Denominator=[0.05 1]
  Kalman8 : TransferFcn  Denominator=[0.05 1]
  MATLAB Function : MATLAB Function  TreatAsAtomicUnit=on
  Mux3 : Mux  Inputs=3
  Mux4 : Mux  Inputs=3
  Mux5 : Mux  Inputs=3
  Sum1 : Sum  Inputs=++|
  Sum3 : Sum  Inputs=++|
  Sum6 : Sum  Inputs=++|
  optitrack_ : Outport  OutDataTypeStr=Bus: BUS_optitrack  VectorParamsAs1DForOutWhenUnconnected=off
  wires:
  Bus Creator/1 -> optitrack_/1
  Delay3/1 -> Sum6/2
  Mux5/1 -> Delay3/1
  Demux11/3 -> Bus Creator/9  "yaw"
  MATLAB Function/1(out) -> Mux5/3
  Demux11/2 -> Bus Creator/8  "Pitch"
  Bus Selector/8 -> Mux5/2  "<Theta>"
  Sum6/1 -> Demux11/1  "angles_mes"
  Demux11/1 -> Bus Creator/7  "roll"
  Band-Limited White Noise5/1 -> Sum6/1
  Bus Selector/7 -> Mux5/1  "<Phi>"
  Sum1/1 -> Demux8/1  "Position_mes"
  Demux8/3 -> Bus Creator/3  "zPos"
  Demux9/2 -> Bus Creator/5  "yVel"
  Demux8/1 -> Bus Creator/1  "xPos"
  Bus Selector/3 -> 1er ordre2/1(z)  "<Z>"
  Demux9/3 -> Bus Creator/6  "zVel"
  1er ordre2/1(z_retard) -> Mux3/3
  Delay7/1 -> Sum1/2
  Demux9/1 -> Bus Creator/4  "xVel"
  Kalman4/1 -> Mux4/3
  Demux8/2 -> Bus Creator/2  "yPos"
  Bus Selector/2 -> 1er ordre1/1(y)  "<Y>"
  1er ordre1/1(y_retard) -> Mux3/2
  Kalman7/1 -> Mux4/1
  Band-Limited White Noise1/1 -> Sum1/1
  Mux4/1 -> Delay1/1
  Bus Selector/1 -> 1er ordre/1(x)  "<X>"
  Sum3/1 -> Demux9/1  "vitesse_Ro_mes"
  1er ordre/1(x_retard) -> Mux3/1
  Delay1/1 -> Sum3/2
  Mux3/1 -> Delay7/1
  Kalman8/1 -> Mux4/2
  Band-Limited White Noise3/1 -> Sum3/1
  pos_att_NED/1 -> Bus Selector/1
  Bus Selector/4 -> Kalman7/1  "<VX>"
  Bus Selector/5 -> Kalman8/1  "<VY>"
  Bus Selector/6 -> Kalman4/1  "<VZ>"
  Bus Selector/9 -> MATLAB Function/1(in)  "<Psi>"

== system SiMoDronesBebopRos_student/OPTITRACK/ROS link + Measure/UDP link ==
  Bus Creator : BusCreator  Inputs=9  OutDataTypeStr=Bus: BUS_optitrack
      settings: InheritFromInputs=off
  Demux : Demux  Outputs=6
  Demux1 : Demux  Outputs=3
  optitrack_pos_vel_uav : Subsystem
  optitrack : Outport  OutDataTypeStr=Bus: BUS_optitrack  VectorParamsAs1DForOutWhenUnconnected=off
  wires:
  Demux1/3 -> Bus Creator/9
  Demux1/2 -> Bus Creator/8
  Demux1/1 -> Bus Creator/7
  Demux/6 -> Bus Creator/6
  Demux/5 -> Bus Creator/5
  Demux/4 -> Bus Creator/4
  Demux/3 -> Bus Creator/3
  Demux/2 -> Bus Creator/2
  Demux/1 -> Bus Creator/1
  Bus Creator/1 -> optitrack/1
  optitrack_pos_vel_uav/2(att_eul_OT) -> Demux1/1
  optitrack_pos_vel_uav/1(pos_vel_OT) -> Demux/1

== system SiMoDronesBebopRos_student/Visu 3D/Simulink 3D/Coordinate Transformations ==
  pos_att_NED : Inport
  Bus Selector : BusSelector  OutputSignals=Phi,Theta,Psi,X,Y,Z
  Gain : Gain  Gain=[1 1 -1 1]
  Gain1 : Gain  Gain=[1 1 -1]
  Gain3 : Gain  Gain=-1
  Math Function : Math  Operator=transpose  SignedPower=on  SaturateOnIntegerOverflow=on
  Mux : Mux  Inputs=3
  Mux2 : Mux  Inputs=3
  Rotation Angles to Direction Cosine Matrix1 : sharedtransform/Rotation Angles to Direction Cosine Matrix  rotationOrder=XYZ  aMode=aMode
      settings: SourceProductBaseCode=AE,PW,DR,MT,UV,VE
  Rotation Matrix to VRML Rotation : vrlib/Utilities/Rotation Matrix to VR Rotation  maxzero=1e-5
      settings: SourceProductBaseCode=SL
  VR Signal Expander : vrlib/VR Signal Expander  outwidth=4  outidx=[1 3 2 4]
  VR Signal Expander1 : vrlib/VR Signal Expander  outwidth=3  outidx=[1 3 2]
  VR Signal Expander2 : vrlib/VR Signal Expander  outwidth=4  outidx=[4]
  CameraFollowRotation : Outport  VectorParamsAs1DForOutWhenUnconnected=off
  CameraFollowTranslation : Outport  Port=2  VectorParamsAs1DForOutWhenUnconnected=off
  orientation : Outport  Port=3  VectorParamsAs1DForOutWhenUnconnected=off
  position : Outport  Port=4  VectorParamsAs1DForOutWhenUnconnected=off
  wires:
  Bus Selector/5 -> Mux2/2  "<Y>"
  Bus Selector/4 -> Mux2/1  "<X>"
  Bus Selector/3 -> Mux/3  "<Psi>"
  Gain3/1 -> VR Signal Expander2/1
  VR Signal Expander2/1 -> CameraFollowRotation/1
  Bus Selector/6 -> Mux2/3, Gain3/1  "<Z>"
  VR Signal Expander1/1 -> CameraFollowTranslation/1, position/1  "pos_VRML"
  Gain/1 -> VR Signal Expander/1
  Rotation Matrix to VRML Rotation/1 -> Gain/1
  Math Function/1 -> Rotation Matrix to VRML Rotation/1  "DCM_Body_2_NED"
  Rotation Angles to Direction Cosine Matrix1/1 -> Math Function/1  "DCM_NED_2_Body"
  Mux/1 -> Rotation Angles to Direction Cosine Matrix1/1
  Gain1/1 -> VR Signal Expander1/1  "pos_ENU"
  Mux2/1 -> Gain1/1  "pos_NED"
  VR Signal Expander/1 -> orientation/1
  pos_att_NED/1 -> Bus Selector/1
  Bus Selector/1 -> Mux/1  "<Phi>"
  Bus Selector/2 -> Mux/2  "<Theta>"

== system SiMoDronesBebopRos_student/BEBOP/Bebop Control/Inner Loop (Parrot)/Bebop onboard control ==
  bebop_tgt : Inport  OutDataTypeStr=Bus: BUS_bebop_tgt
  bebop_ctrl : Inport  Port=2
  bebop_sensors : Inport  Port=3  OutDataTypeStr=Bus: BUS_bebop_sensors
  Bus Creator : BusCreator  Inputs=4  OutDataTypeStr=Bus: BUS_actuator_tgt
  Bus Selector : BusSelector  OutputSignals=Vz
  Bus Selector4 : BusSelector  OutputSignals=roll,pitch,yaw_rate
  Chart : Stateflow chart  TreatAsAtomicUnit=on
  Data Type Conversion : DataTypeConversion
  Régulations : Subsystem
  Saturation : Saturate  UpperLimit=altiVzmax  LowerLimit=-altiVzmax
  Vz control : Subsystem
  actuator_target : Outport  SampleTime=Ts_bebop  VectorParamsAs1DForOutWhenUnconnected=off
  bebop_state : Outport  Port=2  SampleTime=Ts_bebop_feedback  VectorParamsAs1DForOutWhenUnconnected=off
  wires:
  bebop_tgt/1 -> [bebop_tgt], Bus Selector4/1  "att_target_Rb"
  Bus Selector/1 -> Saturation/1  "<Vz>"
  Bus Selector4/2 -> Régulations/2(Theta_c)  "<pitch>"
  Bus Selector4/1 -> Régulations/1(Phi_c)  "<roll>"
  Régulations/1(Out2) -> Bus Creator/1  "roll"
  Régulations/2(Out1) -> Bus Creator/2  "pitch"
  Régulations/3(Cde_R) -> Bus Creator/3  "yaw"
  Vz control/1(thrust) -> Bus Creator/4  "thrust"
  Saturation/1 -> Vz control/1(Vz_d)
  Bus Selector4/3 -> Régulations/3(Cde_Lacet)  "<yaw_rate>"
  bebop_ctrl/1 -> Chart/3(bebop_ctrl)
  [bebop_tgt] -> Bus Selector/1  "att_target_Rb"
  Chart/1(bebop_state) -> bebop_state/1, Vz control/3(bebop_state)  "bebop_state_local"
  bebop_sensors/1 -> Régulations/4(bebop_sensors), Chart/1(bebop_sensors), Vz control/2(bebop_sensor)
  [bebop_tgt] -> Chart/2(bebop_tgt)
  Bus Creator/1 -> actuator_target/1

== system SiMoDronesBebopRos_student/BEBOP/Bebop Control/Inner Loop (Parrot)/Mixer_Quad_X ==
  actuators_tgt : Inport  OutDataTypeStr=Bus: BUS_actuator_tgt
  Bus Selector1 : BusSelector  OutputSignals=roll,pitch,yaw,thrust
  Gain : Gain  Gain=[0.707107 0.707107 -1 1;-0.707107 0.707107 1 1; -0.707107 -0.707107 -1 1; 0.707107 -0.707107 1 1]  Multiplication=Matrix(K*u) (u vector)
  Mux3 : Mux
  pwm_out : Outport  VectorParamsAs1DForOutWhenUnconnected=off  BusOutputAsStruct=on
  wires:
  Mux3/1 -> Gain/1
  actuators_tgt/1 -> Bus Selector1/1
  Bus Selector1/2 -> Mux3/2  "<pitch>"
  Bus Selector1/3 -> Mux3/3  "<yaw>"
  Bus Selector1/1 -> Mux3/1  "<roll>"
  Bus Selector1/4 -> Mux3/4  "<thrust>"
  Gain/1 -> pwm_out/1

== system SiMoDronesBebopRos_student/BEBOP/Bebop Control/Udp send/NED attitude to ENU linear ==
  <pitch> : Inport
  <roll> : Inport  Port=2
  <vz> : Inport  Port=3
  <body_yaw_rate> : Inport  Port=4
  Gain{,1..3} (4 alike) : Gain  Gain=-1
  Gain4 : Gain  Gain=1/controlGains.roll.anglemax
  Gain5 : Gain  Gain=1/controlGains.pitch.anglemax
  Gain6 : Gain  Gain=1/controlGains.psi.ratemax
  Scope : Scope
  Out1 : Outport  VectorParamsAs1DForOutWhenUnconnected=off
  Out2 : Outport  Port=2  VectorParamsAs1DForOutWhenUnconnected=off
  Out3 : Outport  Port=3  VectorParamsAs1DForOutWhenUnconnected=off
  Out4 : Outport  Port=4  VectorParamsAs1DForOutWhenUnconnected=off
  wires:
  Gain3/1 -> Scope/1, Out4/1
  Gain2/1 -> Out3/1
  <roll>/1 -> Gain4/1
  <body_yaw_rate>/1 -> Gain6/1
  <vz>/1 -> Gain2/1
  <pitch>/1 -> Gain5/1
  Gain1/1 -> Out2/1
  Gain/1 -> Out1/1
  Gain5/1 -> Gain/1
  Gain4/1 -> Gain1/1
  Gain6/1 -> Gain3/1

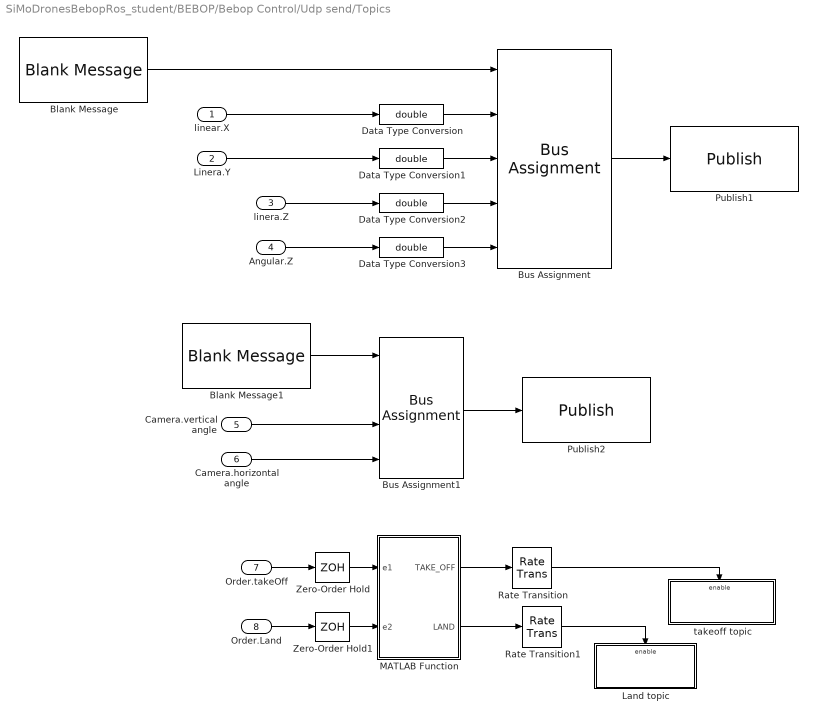
== system SiMoDronesBebopRos_student/BEBOP/Bebop Control/Udp send/Topics ==
  linear.X : Inport
  Linera.Y : Inport  Port=2
  linera.Z : Inport  Port=3
  Angular.Z : Inport  Port=4
  Camera.vertical angle : Inport  Port=5
  Camera.horizontal angle : Inport  Port=6
  Order.takeOff : Inport  Port=7
  Order.Land : Inport  Port=8
  Blank Message : robotlib/Blank Message  messageClass=Message  entityType=geometry_msgs/Twist  messageType=geometry_msgs/Twist  SampleTime=-1  legacyBusStruct=off
  Blank Message1 : robotlib/Blank Message  messageClass=Message  entityType=geometry_msgs/Twist  messageType=geometry_msgs/Twist  SampleTime=-1  legacyBusStruct=off
  Bus Assignment : BusAssignment  AssignedSignals=Linear.X,Linear.Y,Linear.Z,Angular.Z
  Bus Assignment1 : BusAssignment  AssignedSignals=Angular.X,Angular.Y,Angular.Z
  Data Type Conversion{,1..3} (4 alike) : DataTypeConversion  OutDataTypeStr=double
  Land topic : Subsystem  TreatAsAtomicUnit=on
  MATLAB Function : MATLAB Function  TreatAsAtomicUnit=on
  Publish1 : robotlib/Publish  topicSource=Select from ROS network  topic=/bebop/cmd_vel  messageType=geometry_msgs/Twist  legacyBusStruct=off  messageQueueLength=1
  Publish2 : robotlib/Publish  topicSource=Select from ROS network  topic=/bebop/camera_control  messageType=geometry_msgs/Twist  legacyBusStruct=off  messageQueueLength=1
  Rate Transition : RateTransition  OutPortSampleTime=Te_topics_empty
  Rate Transition1 : RateTransition  OutPortSampleTime=Te_topics_empty
  Zero-Order Hold : ZeroOrderHold  SampleTime=5*Te_topics_empty
  Zero-Order Hold1 : ZeroOrderHold  SampleTime=5*Te_topics_empty
  takeoff topic : Subsystem
  wires:
  Bus Assignment/1 -> Publish1/1
  Angular.Z/1 -> Data Type Conversion3/1
  linera.Z/1 -> Data Type Conversion2/1
  linear.X/1 -> Data Type Conversion/1
  Linera.Y/1 -> Data Type Conversion1/1
  Blank Message/1 -> Bus Assignment/1
  Bus Assignment1/1 -> Publish2/1
  Blank Message1/1 -> Bus Assignment1/1
  Camera.vertical angle/1 -> Bus Assignment1/3
  Camera.horizontal angle/1 -> Bus Assignment1/4
  MATLAB Function/1(TAKE_OFF) -> Rate Transition/1
  MATLAB Function/2(LAND) -> Rate Transition1/1
  Data Type Conversion/1 -> Bus Assignment/2
  Data Type Conversion1/1 -> Bus Assignment/3
  Data Type Conversion2/1 -> Bus Assignment/4
  Data Type Conversion3/1 -> Bus Assignment/5
  Order.takeOff/1 -> Zero-Order Hold/1
  Order.Land/1 -> Zero-Order Hold1/1
  Zero-Order Hold/1 -> MATLAB Function/1(e1)
  Zero-Order Hold1/1 -> MATLAB Function/2(e2)
  Rate Transition/1 -> takeoff topic/Enable
  Rate Transition1/1 -> Land topic/Enable

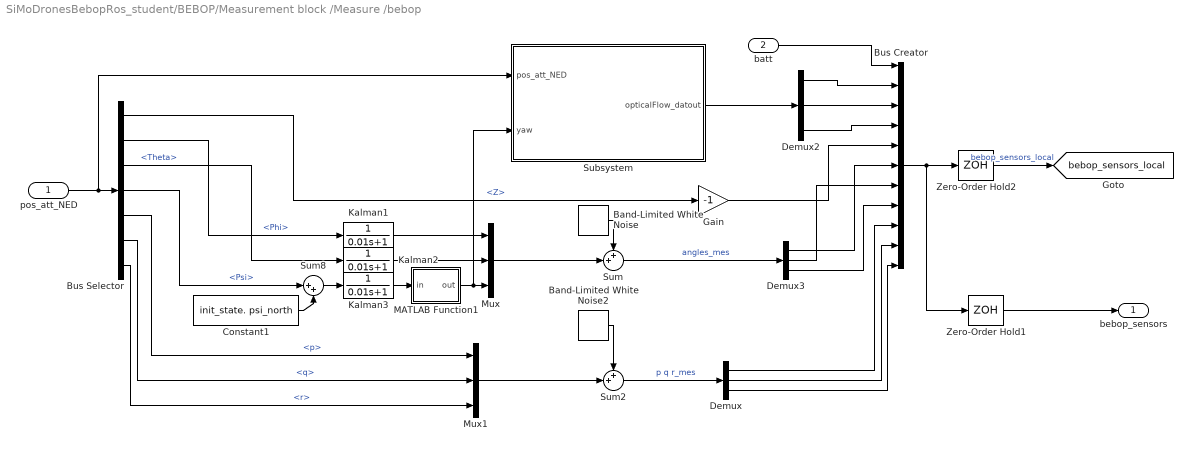
== system SiMoDronesBebopRos_student/BEBOP/Measurement block /Measure /bebop ==
  pos_att_NED : Inport  OutDataTypeStr=Bus: BUS_bebop_pos_att
  batt : Inport  Port=2
  Band-Limited White Noise : simulink/Sources/Band-Limited White Noise  Cov=[measure.noise_power_angles]  Ts=Ts_bebop  seed=[23341]
  Band-Limited White Noise2 : simulink/Sources/Band-Limited White Noise  Cov=[measure.noise_power_pqr]  Ts=Ts_bebop  seed=[23341]
  Bus Creator : BusCreator  Inputs=11  OutDataTypeStr=Bus: BUS_bebop_sensors
      settings: InheritFromInputs=off
  Bus Selector : BusSelector  OutputSignals=Z,Phi,Theta,Psi,p,q,r
  Constant1 : Constant  Value=init_state. psi_north
  Demux : Demux  Outputs=3
  Demux2 : Demux  Outputs=3
  Demux3 : Demux  Outputs=3
  Gain : Gain  Gain=-1
  Kalman1 : TransferFcn  Denominator=[0.01 1]
  Kalman2 : TransferFcn  Denominator=[0.01 1]
  Kalman3 : TransferFcn  Denominator=[0.01 1]
  MATLAB Function1 : MATLAB Function  TreatAsAtomicUnit=on
  Mux : Mux  Inputs=3
  Mux1 : Mux  Inputs=3
  Subsystem : Subsystem
  Sum : Sum  Inputs=++|
  Sum2 : Sum  Inputs=++|
  Sum8 : Sum  Inputs=|++
  Zero-Order Hold1 : ZeroOrderHold  SampleTime=Ts_bebop_feedback
  Zero-Order Hold2 : ZeroOrderHold  SampleTime=Ts_bebop
  bebop_sensors : Outport  OutDataTypeStr=Bus: BUS_bebop_sensors  VectorParamsAs1DForOutWhenUnconnected=off
  tag scope: bebop_sensors_local=global
  wires:
  Bus Selector/4 -> Sum8/1  "<Psi>"
  Sum8/1 -> Kalman3/1
  Constant1/1 -> Sum8/2
  Bus Selector/7 -> Mux1/3  "<r>"
  Mux1/1 -> Sum2/2
  Mux/1 -> Sum/2
  Bus Selector/6 -> Mux1/2  "<q>"
  Bus Selector/5 -> Mux1/1  "<p>"
  Kalman3/1 -> MATLAB Function1/1(in)
  Kalman2/1 -> Mux/2
  Kalman1/1 -> Mux/1
  Bus Selector/3 -> Kalman2/1  "<Theta>"
  Bus Selector/2 -> Kalman1/1  "<Phi>"
  Band-Limited White Noise2/1 -> Sum2/1
  Band-Limited White Noise/1 -> Sum/1
  Sum/1 -> Demux3/1  "angles_mes"
  Bus Selector/1 -> Gain/1  "<Z>"
  MATLAB Function1/1(out) -> Subsystem/2(yaw), Mux/3
  batt/1 -> Bus Creator/1
  Subsystem/1(opticalFlow_datout) -> Demux2/1
  Demux2/1 -> Bus Creator/2
  Demux2/2 -> Bus Creator/3
  Demux2/3 -> Bus Creator/4
  Demux3/3 -> Bus Creator/8
  Demux3/2 -> Bus Creator/7
  Demux3/1 -> Bus Creator/6
  Sum2/1 -> Demux/1  "p q r_mes"
  Bus Creator/1 -> Zero-Order Hold2/1, Zero-Order Hold1/1
  Zero-Order Hold1/1 -> bebop_sensors/1
  Zero-Order Hold2/1 -> [bebop_sensors_local]  "bebop_sensors_local"
  pos_att_NED/1 -> Subsystem/1(pos_att_NED), Bus Selector/1
  Gain/1 -> Bus Creator/5
  Demux/3 -> Bus Creator/11
  Demux/2 -> Bus Creator/10
  Demux/1 -> Bus Creator/9

== system SiMoDronesBebopRos_student/BEBOP/Measurement block /ROS link + Measure/UDP link ==
  Bus Creator1 : BusCreator  Inputs=11  OutDataTypeStr=Bus: BUS_bebop_sensors
      settings: InheritFromInputs=off
  Bus Selector : BusSelector  OutputSignals=X,Y,Z
  Bus Selector1 : BusSelector  OutputSignals=Data
  Bus Selector2 : BusSelector  OutputSignals=Linear.X,Linear.Y,Linear.Z
  Bus Selector3 : BusSelector  OutputSignals=Data
  Constant : Constant  Value=0  SampleTime=Ts_bebop_feedback
  Constant1 : Constant  Value=0  SampleTime=Ts_bebop_feedback
  Constant2 : Constant  Value=0  SampleTime=Ts_bebop_feedback
  "ENU bebop -> NED" : Subsystem
  Subscribe : robotlib/Subscribe  topicSource=Select from ROS network  topic=/bebop/attitude  messageType=geometry_msgs/Vector3  SampleTime=Ts_bebop_feedback  legacyBusStruct=off  messageQueueLength=1
  Subscribe1 : robotlib/Subscribe  topicSource=Select from ROS network  topic=/bebop/battery  messageType=std_msgs/Float64  SampleTime=Ts_bebop_feedback  legacyBusStruct=off  messageQueueLength=1
  Subscribe2 : robotlib/Subscribe  topicSource=Select from ROS network  topic=/bebop/speed  messageType=geometry_msgs/Twist  SampleTime=Ts_bebop_feedback  legacyBusStruct=off  messageQueueLength=1
  Subscribe3 : robotlib/Subscribe  topicSource=Select from ROS network  topic=/bebop/altitude  messageType=std_msgs/Float64  SampleTime=Ts_bebop_feedback  legacyBusStruct=off  messageQueueLength=1
  Terminator{,1..3} (4 alike) : Terminator
  bebop_sensors : Outport  OutDataTypeStr=Bus: BUS_bebop_sensors  VectorParamsAs1DForOutWhenUnconnected=off
  wires:
  Bus Selector/1 -> "ENU bebop -> NED"/1(<X>)  "<X>"
  Subscribe1/2 -> Bus Selector1/1
  Subscribe/2 -> Bus Selector/1
  Bus Selector/2 -> "ENU bebop -> NED"/2(<Y>)  "<Y>"
  Subscribe2/2 -> Bus Selector2/1
  Subscribe3/2 -> Bus Selector3/1
  Bus Selector/3 -> "ENU bebop -> NED"/3(<Z>)  "<Z>"
  Bus Creator1/1 -> bebop_sensors/1
  Bus Selector1/1 -> Bus Creator1/1  "<Data>"
  Bus Selector2/3 -> Bus Creator1/4  "<Z>"
  Bus Selector2/2 -> Bus Creator1/3  "<Y>"
  Bus Selector2/1 -> Bus Creator1/2  "<X>"
  Bus Selector3/1 -> Bus Creator1/5  "<Data>"
  "ENU bebop -> NED"/3(Out3) -> Bus Creator1/8
  "ENU bebop -> NED"/2(Out2) -> Bus Creator1/7
  "ENU bebop -> NED"/1(Out1) -> Bus Creator1/6
  Subscribe1/1 -> Terminator/1
  Subscribe2/1 -> Terminator1/1
  Subscribe3/1 -> Terminator2/1
  Subscribe/1 -> Terminator3/1
  Constant/1 -> Bus Creator1/9
  Constant1/1 -> Bus Creator1/10
  Constant2/1 -> Bus Creator1/11

== system SiMoDronesBebopRos_student/BEBOP/Model/Model/Acutators1 ==
  pwm_target : Inport
  Demux : Demux
  Motor1 : Subsystem
  Motor2 : Subsystem
  Motor3 : Subsystem
  Motor4 : Subsystem
  Mux : Mux
  prop speed [rad/s] : Outport  VectorParamsAs1DForOutWhenUnconnected=off
  wires:
  pwm_target/1 -> Demux/1
  Mux/1 -> prop speed [rad/s]/1
  Demux/1 -> Motor1/1(PWM)
  Demux/4 -> Motor4/1(PWM)
  Demux/3 -> Motor3/1(PWM)
  Demux/2 -> Motor2/1(PWM)
  Motor3/1(speed) -> Mux/3
  Motor4/1(speed) -> Mux/4
  Motor2/1(speed) -> Mux/2
  Motor1/1(speed) -> Mux/1
